simulink library "dspilbclib"  (Simulink 8.3)
settings: Solver=ode45  SolverMode=SingleTasking  StartTime=0.0  StopTime=10.0  RelTol=1e-3
undefined symbols (not defined in the file or in its folder): dfilt, ilbc, ilbcMode
libraries: dspsigops x6, dspmtrx3 x4, dspquant2 x3, dsparch4 x2, dspilbclib x1, dsplp x1
settings Model: Creator=The MathWorks Inc.  ExtModeAutoUpdateStatusClock=off

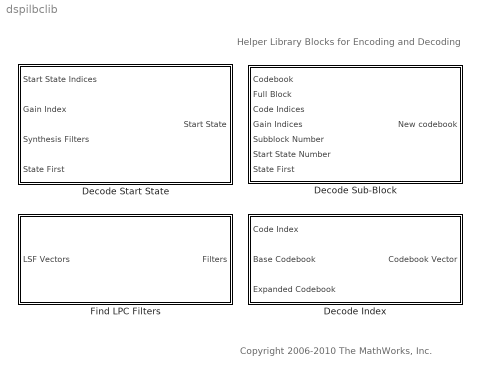
== system dspilbclib ==
  note: Helper Library Blocks for Encoding and Decoding
  note: Copyright 2006-2010 The MathWorks, Inc.
  Decode Index : Subsystem  TreatAsAtomicUnit=on
  Decode Start State : Subsystem  TreatAsAtomicUnit=on
  Decode Sub-Block : Subsystem  TreatAsAtomicUnit=on
  Find LPC Filters : Subsystem  TreatAsAtomicUnit=on

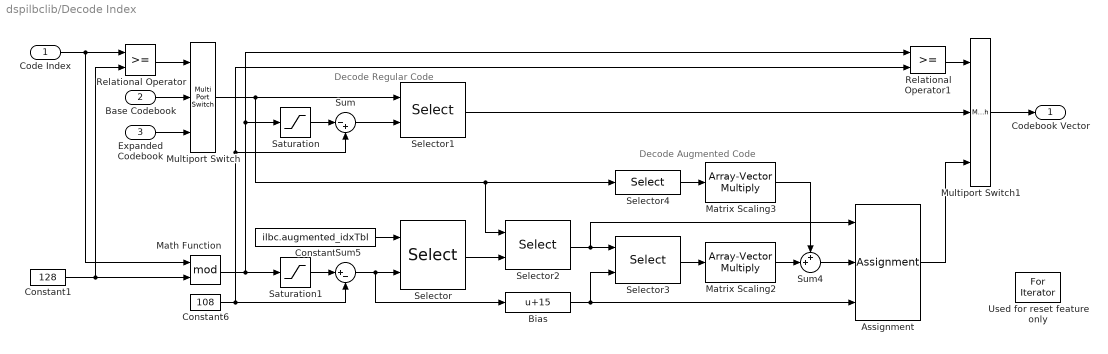
== system dspilbclib/Decode Index ==
  note: Decode Regular Code
  note: Decode Augmented Code
  Code Index : Inport
  Base Codebook : Inport  Port=2
  Expanded Codebook : Inport  Port=3
  Assignment : Assignment  NumberOfDimensions=2  IndexMode=Zero-based  IndexOptions=Starting index (port),Assign all  Indices=1,1  OutputSizes=40,1
  Bias : Bias  Bias=15
  Constant : Constant  Value=ilbc.augmented_idxTbl  VectorParams1D=off  OutDataTypeStr=uint8
  Constant1 : Constant  Value=128  OutDataTypeStr=uint8
  Constant6 : Constant  Value=108  OutDataTypeStr=uint8
  Math Function : Math  Operator=mod  SaturateOnIntegerOverflow=on
  Matrix Scaling2 : dspmtrx3/Array-Vector Multiply  mode=Mute  saveAsFlag=0  Dimension=1  V_Source=Dialog parameter  V_VectFromMask=[0 0.2 0.4 0.6 0.8]  firstCoeffSignedness=Auto  firstCoeffDataTypeStr=Inherit: Same word length as input  firstCoeffLastDataTypeStr=Inherit: Same word length as input  firstCoeffMin=[]  firstCoeffMax=[]  outputSignedness=Auto  outputDataTypeStr=Inherit: Same as product output  outputLastDataTypeStr=Inherit: Same as product output  outputMin=[]  outputMax=[]  accumSignedness=Auto  prodOutputSignedness=Auto  roundingMode=Floor  overflowMode=off
  Matrix Scaling3 : dspmtrx3/Array-Vector Multiply  mode=Mute  saveAsFlag=0  Dimension=1  V_Source=Dialog parameter  V_VectFromMask=[1 0.8 0.6 0.4 0.2]  firstCoeffSignedness=Auto  firstCoeffDataTypeStr=Inherit: Same word length as input  firstCoeffLastDataTypeStr=Inherit: Same word length as input  firstCoeffMin=[]  firstCoeffMax=[]  outputSignedness=Auto  outputDataTypeStr=Inherit: Same as product output  outputLastDataTypeStr=Inherit: Same as product output  outputMin=[]  outputMax=[]  accumSignedness=Auto  prodOutputSignedness=Auto  roundingMode=Floor  overflowMode=off
  Multiport Switch : MultiPortSwitch  DataPortOrder=Zero-based contiguous  Inputs=2  zeroidx=on
  Multiport Switch1 : MultiPortSwitch  DataPortOrder=Zero-based contiguous  Inputs=2  zeroidx=on
  Relational Operator : RelationalOperator  OutDataTypeStr=boolean
  Relational Operator1 : RelationalOperator  OutDataTypeStr=boolean
  Saturation : Saturate  UpperLimit=107  LowerLimit=0
  Saturation1 : Saturate  UpperLimit=127  LowerLimit=108
  Selector : Selector  NumberOfDimensions=2  IndexMode=Zero-based  InputPortWidth=3  IndexOptions=Select all,Index vector (port)  Indices=[1 3],1  OutputSizes=1,1
  Selector1 : Selector  NumberOfDimensions=2  InputPortWidth=3  IndexOptions=Starting index (port),Select all  Indices=1,-1  OutputSizes=40,1
  Selector2 : Selector  NumberOfDimensions=2  InputPortWidth=3  IndexOptions=Index vector (port),Select all  Indices=[1 3],1  OutputSizes=1,1
  Selector3 : Selector  NumberOfDimensions=2  IndexMode=Zero-based  InputPortWidth=3  IndexOptions=Starting index (port),Select all  Indices=[1 3],1  OutputSizes=5,5
  Selector4 : Selector  NumberOfDimensions=2  InputPortWidth=3  IndexOptions=Index vector (dialog),Select all  Indices=[143:147],1  OutputSizes=1,1
  Sum : Sum  Inputs=|-+
  Sum4 : Sum  Inputs=++|
  Sum5 : Sum  Inputs=|+-
  Used for reset feature only : ForIterator  ResetStates=reset  IterationLimit=1  ShowIterationPort=off  IterationVariableDataType=int8
  Codebook Vector : Outport
  wires:
  Base Codebook/1 -> Multiport Switch/2
  Multiport Switch/1 -> Selector1/1, Selector4/1, Selector2/1
  Expanded Codebook/1 -> Multiport Switch/3
  Sum/1 -> Selector1/2
  Relational Operator1/1 -> Multiport Switch1/1
  Multiport Switch1/1 -> Codebook Vector/1
  Selector1/1 -> Multiport Switch1/2
  Saturation/1 -> Sum/1
  Constant6/1 -> Sum5/2, Sum/2, Relational Operator1/2
  Saturation1/1 -> Sum5/1
  Math Function/1 -> Saturation1/1, Saturation/1, Relational Operator1/1
  Constant1/1 -> Math Function/2, Relational Operator/2
  Relational Operator/1 -> Multiport Switch/1
  Code Index/1 -> Relational Operator/1, Math Function/1
  Sum5/1 -> Selector/2, Bias/1
  Selector3/1 -> Matrix Scaling2/1
  Selector2/1 -> Selector3/1, Assignment/1
  Selector/1 -> Selector2/2
  Constant/1 -> Selector/1
  Matrix Scaling2/1 -> Sum4/2
  Selector4/1 -> Matrix Scaling3/1
  Matrix Scaling3/1 -> Sum4/1
  Sum4/1 -> Assignment/2
  Bias/1 -> Selector3/2, Assignment/3
  Assignment/1 -> Multiport Switch1/3

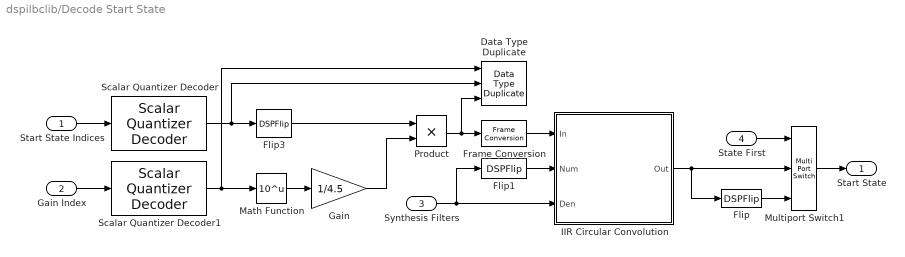
== system dspilbclib/Decode Start State ==
  Start State Indices : Inport
  Gain Index : Inport  Port=2
  Synthesis Filters : Inport  Port=3
  State First : Inport  Port=4
  Data Type Duplicate : DataTypeDuplicate  NumInputPorts=3
  Flip : DSPFlip
  Flip1 : DSPFlip
  Flip3 : DSPFlip
  Frame Conversion : FrameConversion
  Gain : Gain  Gain=1/4.5  OutDataTypeStr=Inherit: Inherit via back propagation
  IIR Circular Convolution : Subsystem  TreatAsAtomicUnit=on
  Math Function : Math  Operator=10^u  SaturateOnIntegerOverflow=on
  Multiport Switch1 : MultiPortSwitch  DataPortOrder=Zero-based contiguous  Inputs=2  zeroidx=on
  Product : Product  OutDataTypeStr=Inherit: Inherit via back propagation  RndMeth=Zero
  Scalar Quantizer Decoder : dspquant2/Scalar Quantizer Decoder  invalidin=Clip  CBsource=Specify via dialog  codebook=ilbc.state_sq3Tbl  dataType=Inherit via back propagation  isSigned=on  wordLen=16  udDataType=sfix(16)  fracBitsMode=Best precision  numFracBits=11  OutDataTypeStr=Inherit: Inherit via back propagation  LastOutDataTypeStr=Inherit: Inherit via back propagation
  Scalar Quantizer Decoder1 : dspquant2/Scalar Quantizer Decoder  invalidin=Clip  CBsource=Specify via dialog  codebook=ilbc.state_frgqTbl  dataType=Inherit via back propagation  isSigned=on  wordLen=16  udDataType=}  fracBitsMode=Best precision  numFracBits=11  OutDataTypeStr=Inherit: Inherit via back propagation  LastOutDataTypeStr=Inherit: Inherit via back propagation
  Start State : Outport
  wires:
  Gain Index/1 -> Scalar Quantizer Decoder1/1
  Scalar Quantizer Decoder1/1 -> Math Function/1, Data Type Duplicate/1
  Start State Indices/1 -> Scalar Quantizer Decoder/1
  Scalar Quantizer Decoder/1 -> Flip3/1, Data Type Duplicate/2
  Flip1/1 -> IIR Circular Convolution/2(Num)
  Synthesis Filters/1 -> Flip1/1, IIR Circular Convolution/3(Den)
  Product/1 -> Frame Conversion/1, Data Type Duplicate/3
  IIR Circular Convolution/1(Out) -> Multiport Switch1/2, Flip/1
  Math Function/1 -> Gain/1
  Frame Conversion/1 -> IIR Circular Convolution/1(In)
  Flip/1 -> Multiport Switch1/3
  State First/1 -> Multiport Switch1/1
  Multiport Switch1/1 -> Start State/1
  Gain/1 -> Product/2
  Flip3/1 -> Product/1

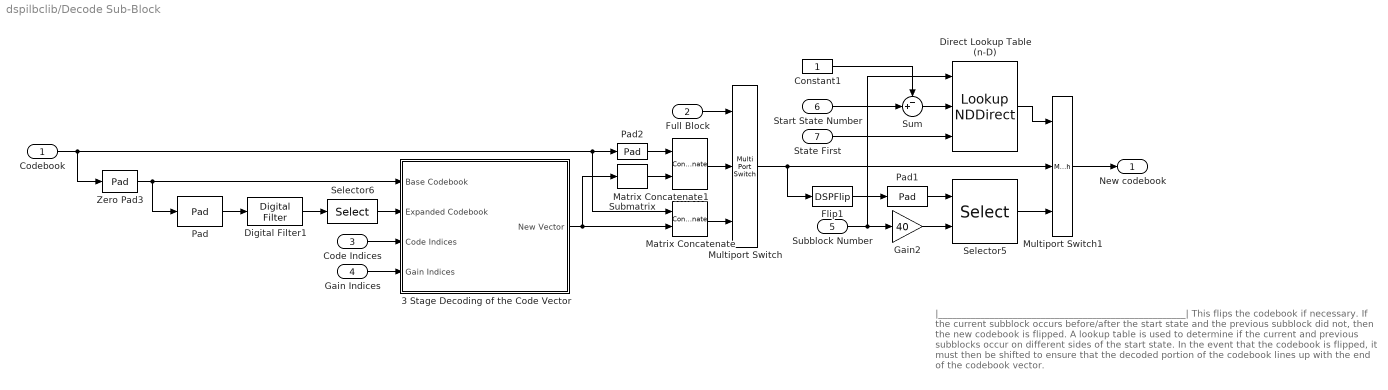
== system dspilbclib/Decode Sub-Block ==
  note: |_____________________________________________________|
      |
      | This flips the codebook if necessary.  If the current subblock occurs before/after the start
      | state and the previous subblock did not, then the new codebook is flipped.  A lookup table
      | is used to determine if the current and previous subblocks occur on different sides of
      | the start state.  In the event that the codebook is flipped, it must then be shifted to ensure
      | that the decoded portion of the codebook lines up with the end of the codebook vector.
  Codebook : Inport
  Full Block : Inport  Port=2
  Code Indices : Inport  Port=3
  Gain Indices : Inport  Port=4
  Subblock Number : Inport  Port=5
  Start State Number : Inport  Port=6
  State First : Inport  Port=7
  3 Stage Decoding of the Code Vector : Subsystem  TreatAsAtomicUnit=on
  Constant1 : Constant  OutDataTypeStr=uint8
  Digital Filter1 : dsparch4/Digital Filter  TypePopup=FIR (all zeros)  IIRFiltStruct=Direct form II transposed  AllPoleFiltStruct=Direct form  FIRFiltStruct=Direct form  CoeffSource=Specify via dialog  NumCoeffs=ilbc.cbfiltersTbl  DenCoeffs=[-0.034180 0.108887 -0.184326 0.806152 0.713379 -0.144043 0.083740 -0.033691]  BiQuadCoeffs=[1 0.3 0.4 1 0.1 0.2]  LatticeCoeffs=[0.2 0.4]  denIgnore=on  FiltPerSampPopup=One filter per frame  IC=0  ICnum=0  ICden=0  roundingMode=Floor  overflowMode=off  ScaleValues=1  scaleValueFracLength=14  stageInFracLength=15  stageOutFracLength=15  FilterSource=Specify via dialog  dfiltObjectName=dfilt.dffir([1 2 1])  InputProcessing=Columns as channels (frame based)
  Direct Lookup Table (n-D) : LookupNDDirect  NumberOfTableDimensions=3  Table=ilbc.flip_subblockTbl{ilbcMode}
  Flip1 : DSPFlip
  Gain2 : Gain  Gain=40  OutDataTypeStr=Inherit: Same as input
  Matrix Concatenate : Concatenate  Mode=Multidimensional array
  Matrix Concatenate1 : Concatenate  Mode=Multidimensional array
  Multiport Switch : MultiPortSwitch  DataPortOrder=Zero-based contiguous  Inputs=2  zeroidx=on
  Multiport Switch1 : MultiPortSwitch  DataPortOrder=Zero-based contiguous  Inputs=2  zeroidx=on
  Pad : dspsigops/Pad  padAlong=Specified dimensions  dimsToPad=1  valSrc=Specify via dialog  padVal=0  spec=Pad size  padNumOutRowsSpecMethod=User-specified  numOutRows=1  padNumOutColsSpecMethod=User-specified  numOutCols=1  isVarDimsMode=off  padBeginning=4  padEnd=4  outSizeMode=User-specified  outSize=1  padSigAt=End  trunc_flag=None  roundingMode=Floor  overflowMode=off  truncOrWrapMode=Truncate  wrap_flag=None
  Pad1 : dspsigops/Pad  padAlong=Columns  dimsToPad=1  valSrc=Specify via dialog  padVal=0  spec=Pad size  padNumOutRowsSpecMethod=User-specified  numOutRows=2*ilbc.BLOCKL{ilbcMode}-80  padNumOutColsSpecMethod=User-specified  numOutCols=1  isVarDimsMode=off  padBeginning=0  padEnd=0  outSizeMode=User-specified  outSize=1  padSigAt=Beginning  trunc_flag=None  roundingMode=Floor  overflowMode=off  truncOrWrapMode=Truncate  wrap_flag=None
  Pad2 : dspsigops/Pad  padAlong=Columns  dimsToPad=1  valSrc=Specify via dialog  padVal=0  spec=Output size  padNumOutRowsSpecMethod=User-specified  numOutRows=ilbc.BLOCKL{ilbcMode}-(80-ilbc.STATE_SHORT_LEN{ilbcMode})  padNumOutColsSpecMethod=User-specified  numOutCols=1  isVarDimsMode=off  padBeginning=0  padEnd=80  outSizeMode=User-specified  outSize=1  padSigAt=Beginning  trunc_flag=None  roundingMode=Floor  overflowMode=off  truncOrWrapMode=Truncate  wrap_flag=None
  Selector5 : Selector  NumberOfDimensions=2  IndexMode=Zero-based  InputPortWidth=3  IndexOptions=Starting index (port),Select all  Indices=1:240,1  OutputSizes=ilbc.BLOCKL{ilbcMode},1
  Selector6 : Selector  NumberOfDimensions=2  InputPortWidth=3  IndexOptions=Index vector (dialog),Select all  Indices=9:155,-1
  Submatrix : dspmtrx3/Submatrix  RowSpan=Range of rows  RowStartMode=Offset from last  RowStartIndex=80-ilbc.STATE_SHORT_LEN{ilbcMode}-1  RowEndMode=Last  RowEndIndex=1  ColSpan=All columns  ColStartMode=First  ColStartIndex=1  ColEndMode=Last  ColEndIndex=1
  Sum : Sum  Inputs=-+|
  Zero Pad3 : dspsigops/Pad  padAlong=Columns  dimsToPad=1  valSrc=Specify via dialog  padVal=0  spec=Output size  padNumOutRowsSpecMethod=User-specified  numOutRows=147  padNumOutColsSpecMethod=User-specified  numOutCols=1  isVarDimsMode=off  padBeginning=0  padEnd=0  outSizeMode=User-specified  outSize=1  padSigAt=Beginning  trunc_flag=None  roundingMode=Floor  overflowMode=off  truncOrWrapMode=Truncate  wrap_flag=None
  New codebook : Outport
  wires:
  Codebook/1 -> Matrix Concatenate/1, Pad2/1, Zero Pad3/1
  Pad2/1 -> Matrix Concatenate1/1
  Submatrix/1 -> Matrix Concatenate1/2
  Matrix Concatenate1/1 -> Multiport Switch/2
  Matrix Concatenate/1 -> Multiport Switch/3
  Multiport Switch/1 -> Multiport Switch1/2, Flip1/1
  Gain Indices/1 -> 3 Stage Decoding of the Code Vector/4(Gain Indices)
  Full Block/1 -> Multiport Switch/1
  Code Indices/1 -> 3 Stage Decoding of the Code Vector/3(Code Indices)
  Selector5/1 -> Multiport Switch1/3
  Flip1/1 -> Pad1/1
  Gain2/1 -> Selector5/2
  Pad1/1 -> Selector5/1
  Multiport Switch1/1 -> New codebook/1
  Subblock Number/1 -> Gain2/1, Direct Lookup Table (n-D)/1
  State First/1 -> Direct Lookup Table (n-D)/3
  Direct Lookup Table (n-D)/1 -> Multiport Switch1/1
  3 Stage Decoding of the Code Vector/1(New Vector) -> Matrix Concatenate/2, Submatrix/1
  Sum/1 -> Direct Lookup Table (n-D)/2
  Constant1/1 -> Sum/1
  Start State Number/1 -> Sum/2
  Pad/1 -> Digital Filter1/1
  Digital Filter1/1 -> Selector6/1
  Zero Pad3/1 -> 3 Stage Decoding of the Code Vector/1(Base Codebook), Pad/1
  Selector6/1 -> 3 Stage Decoding of the Code Vector/2(Expanded Codebook)

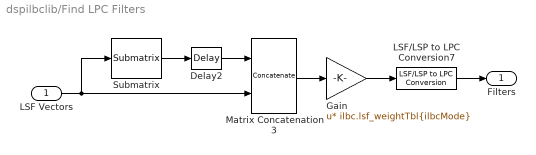
== system dspilbclib/Find LPC Filters ==
  LSF Vectors : Inport
  Delay2 : dspsigops/Delay  InputProcessing=Columns as channels (frame based)  dly_unit=Frames  delay=1  ic_detail=off  dif_ic_for_ch=off  dif_ic_for_dly=on  ic=ilbc.lsfmeanTbl  reset_popup=None
  Gain : Gain  Gain=ilbc.lsf_weightTbl{ilbcMode}  Multiplication=Matrix(u*K)  OutDataTypeStr=Inherit: Same as input  ParamDataTypeStr=Inherit: Same as input
  LSF/LSP to LPC Conversion7 : dsplp/LSF//LSP to LPC Conversion  input=LSF in range (0 pi)
  Matrix Concatenation3 : Concatenate  Mode=Multidimensional array  ConcatenateDimension=2
  Submatrix : dspmtrx3/Submatrix  RowSpan=All rows  RowStartMode=First  RowStartIndex=1  RowEndMode=Last  RowEndIndex=1  ColSpan=Range of columns  ColStartMode=Last  ColStartIndex=1  ColEndMode=Last  ColEndIndex=1
  Filters : Outport
  wires:
  LSF/LSP to LPC Conversion7/1 -> Filters/1
  LSF Vectors/1 -> Submatrix/1, Matrix Concatenation3/2
  Submatrix/1 -> Delay2/1
  Delay2/1 -> Matrix Concatenation3/1
  Gain/1 -> LSF/LSP to LPC Conversion7/1
  Matrix Concatenation3/1 -> Gain/1

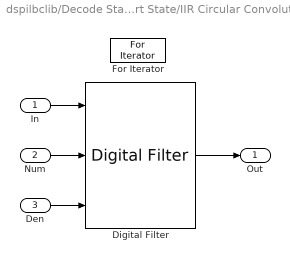
== system dspilbclib/Decode Start State/IIR Circular Convolution ==
  In : Inport
  Num : Inport  Port=2
  Den : Inport  Port=3
  Digital Filter : dsparch4/Digital Filter  TypePopup=IIR (poles & zeros)  IIRFiltStruct=Direct form II transposed  AllPoleFiltStruct=Direct form  FIRFiltStruct=Direct form  CoeffSource=Input port(s)  NumCoeffs=[1 2]  DenCoeffs=[1 0.1]  BiQuadCoeffs=[1 0.3 0.4 1 0.1 0.2]  LatticeCoeffs=[0.2 0.4]  denIgnore=on  FiltPerSampPopup=One filter per frame  IC=0  ICnum=0  ICden=0  roundingMode=Floor  overflowMode=off  ScaleValues=1  scaleValueFracLength=14  stageInFracLength=15  stageOutFracLength=15  FilterSource=Input port(s)  dfiltObjectName=dfilt.dffir([1 2 1])  InputProcessing=Columns as channels (frame based)
  For Iterator : ForIterator  ResetStates=reset  IterationLimit=2  ShowIterationPort=off
  Out : Outport
  wires:
  Den/1 -> Digital Filter/3
  Num/1 -> Digital Filter/2
  In/1 -> Digital Filter/1
  Digital Filter/1 -> Out/1

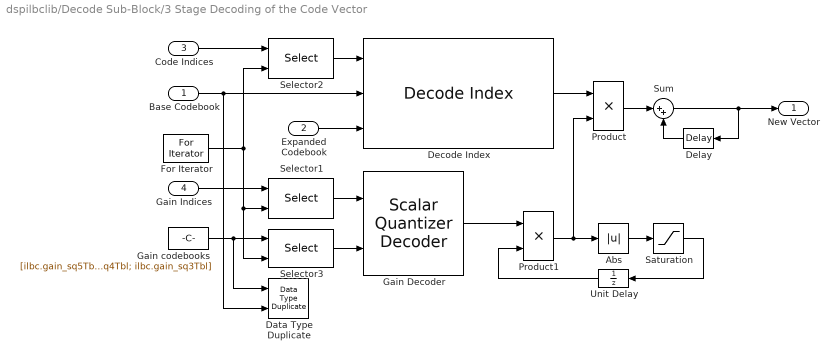
== system dspilbclib/Decode Sub-Block/3 Stage Decoding of the Code Vector ==
  Base Codebook : Inport
  Expanded Codebook : Inport  Port=2
  Code Indices : Inport  Port=3
  Gain Indices : Inport  Port=4
  Abs : Abs
  Data Type Duplicate : DataTypeDuplicate
  Decode Index : dspilbclib/Decode Index
  Delay : dspsigops/Delay  InputProcessing=Columns as channels (frame based)  dly_unit=Frames  delay=1  ic_detail=off  dif_ic_for_ch=off  dif_ic_for_dly=off  ic=0  reset_popup=None
  For Iterator : ForIterator  ResetStates=reset  IterationLimit=3  IndexMode=Zero-based
  Gain codebooks : Constant  Value=[ilbc.gain_sq5Tbl; ilbc.gain_sq4Tbl; ilbc.gain_sq3Tbl]  VectorParams1D=off  OutDataTypeStr=Inherit: Inherit via back propagation
  Gain Decoder : dspquant2/Scalar Quantizer Decoder  invalidin=Clip  CBsource=Input port  codebook=ilbc.gain_sq5Tbl  dataType=User-defined  isSigned=on  wordLen=16  udDataType=float('single')  fracBitsMode=Best precision  numFracBits=11  OutDataTypeStr=double  LastOutDataTypeStr=double
  Product : Product  RndMeth=Zero
  Product1 : Product  RndMeth=Zero
  Saturation : Saturate  UpperLimit=inf  LowerLimit=0.1
  Selector1 : Selector  NumberOfDimensions=2  IndexMode=Zero-based  InputPortWidth=3  IndexOptions=Index vector (port),Select all  Indices=1,1  OutputSizes=1,1
  Selector2 : Selector  NumberOfDimensions=2  IndexMode=Zero-based  InputPortWidth=3  IndexOptions=Index vector (port),Select all  Indices=1,1  OutputSizes=1,1
  Selector3 : Selector  NumberOfDimensions=2  IndexMode=Zero-based  InputPortWidth=3  IndexOptions=Index vector (port),Select all  Indices=1,1  OutputSizes=1,1
  Sum : Sum  Inputs=|++
  Unit Delay : UnitDelay  InitialCondition=1  SampleTime=-1
  New Vector : Outport
  wires:
  Selector2/1 -> Decode Index/1
  Code Indices/1 -> Selector2/1
  Base Codebook/1 -> Decode Index/2, Data Type Duplicate/2
  Expanded Codebook/1 -> Decode Index/3
  Abs/1 -> Saturation/1
  Decode Index/1 -> Product/1
  Product/1 -> Sum/1
  Gain Decoder/1 -> Product1/1
  Product1/1 -> Abs/1, Product/2
  Saturation/1 -> Unit Delay/1
  Selector1/1 -> Gain Decoder/1
  Gain Indices/1 -> Selector1/1
  Selector3/1 -> Gain Decoder/2
  Unit Delay/1 -> Product1/2
  Sum/1 -> New Vector/1, Delay/1
  Delay/1 -> Sum/2
  For Iterator/1 -> Selector3/2, Selector1/2, Selector2/2
  Gain codebooks/1 -> Selector3/1, Data Type Duplicate/1
